simulink model "pigeon_rb300_exec"  (Simulink 3.00)
libraries: execlib x5

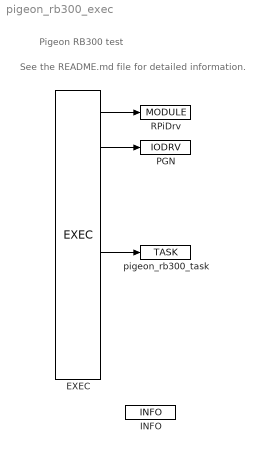
== system pigeon_rb300_exec ==
  note: See the README.md file for detailed information.
  note: Pigeon RB300 test
  EXEC : execlib/EXEC  target=Generic target device  tick=0.001  ntick0=1  ntick1=50  ntick2=100  ntick3=1200  pri0=5  pri1=9  pri2=13  pri3=18
  INFO : execlib/INFO  Title=Pigeon PLC - Simple PID loop  Author=REX Controls s.r.o.  Description=A simple PID feedback control loop on Pigeon RB300  Customer=Users of the REX Control System
  PGN : execlib/IODRV  module=RPiDrv  classname=PgnDrv  factor=1  stack=10240  pri=3  timer=off
  RPiDrv : execlib/MODULE
  pigeon_rb300_task : execlib/TASK  factor=1  start=0  stop=1  stack=10240  MDLOPEN=on
  wires:
  EXEC/1 -> RPiDrv/1
  EXEC/2 -> PGN/1
  EXEC/5 -> pigeon_rb300_task/1
